simulink model "adaptive_mpc_simulink"  (R2019a)
settings: Solver=VariableStepAuto  StartTime=0.0  StopTime=10.0  RelTol=1e-3
libraries: mpclib x1
settings Model: Creator=alexh  LastModifiedBy=alexh

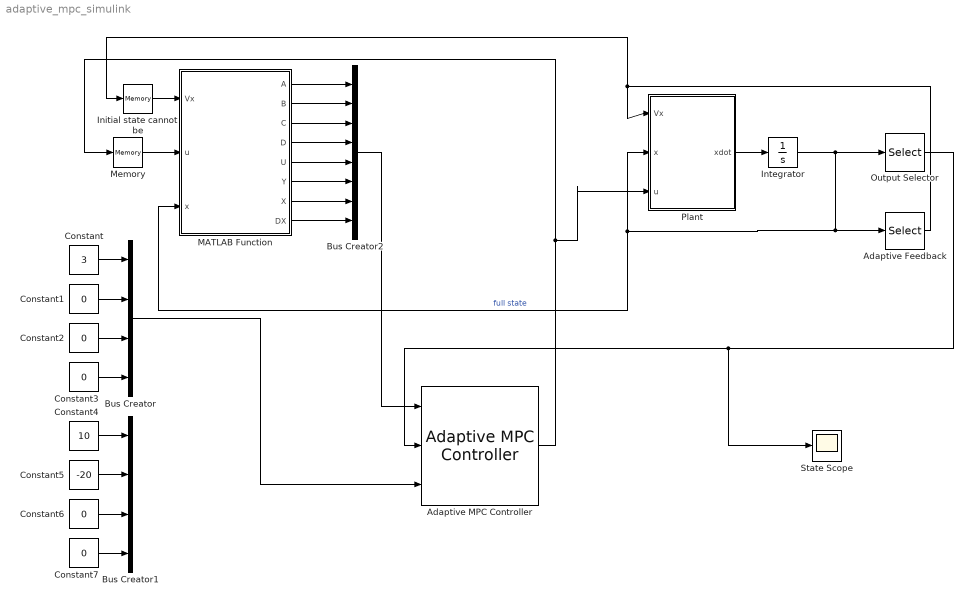
== system adaptive_mpc_simulink ==
  Adaptive Feedback : Selector  InputPortWidth=6  IndexOptions=Index vector (dialog)  Indices=[6]  OutputSizes=1
  Adaptive MPC Controller : mpclib/Adaptive MPC Controller  SCDEnableBlockLinearizationSpecification=on  mpcobj=mpc1_1_C  enable_value=0  updateMPCinCallerWorkspace=on  md_inport=off  mv_inport=off  uref_inport=off  return_cost=off  return_mvseq=off  return_qpstatus=off  return_xseq=off  return_state=off  return_ovseq=off  state_inport=off  isltv_plant=off  umin_inport=off  umax_inport=off  ymin_inport=off  ymax_inport=off  cc_inport=off  ywt_inport=off  uwt_inport=off  duwt_inport=off  rhoeps_inport=off  pm_inport=off  MaximumP=10  HorizonChoice=FixedHorizon  BlockDataType=double  SampleTimeInherited=off  switch_inport=off
      settings: SourceProductName=MATLAB Runtime - Model Predictive Control Toolbox Addin  SourceProductBaseCode=Missing
  Bus Creator : BusCreator  Inputs=4
  Bus Creator1 : BusCreator  Inputs=4
  Bus Creator2 : BusCreator  Inputs=8
  Constant : Constant  Value=3
  Constant{1..3,6..7} (5 alike) : Constant  Value=0
  Constant4 : Constant  Value=10
  Constant5 : Constant  Value=-20
  "Initial state cannot be " : Memory  InitialCondition=1
  Integrator : Integrator  ContinuousStateAttributes='vehicleState'
  MATLAB Function : MATLAB Function  TreatAsAtomicUnit=on
  Memory : Memory
  Output Selector : Selector  InputPortWidth=6  IndexOptions=Index vector (dialog)  Indices=[1 2 3 6]  OutputSizes=1
  Plant : MATLAB Function  TreatAsAtomicUnit=on
  State Scope : Scope
  wires:
  Adaptive MPC Controller/1 -> Memory/1, Plant/3(u)
  Plant/1(xdot) -> Integrator/1
  Integrator/1 -> Output Selector/1, Plant/2(x), MATLAB Function/3(x), Adaptive Feedback/1  "full state"
  Output Selector/1 -> State Scope/1, Adaptive MPC Controller/2
  Constant/1 -> Bus Creator/1
  Constant1/1 -> Bus Creator/2
  Constant2/1 -> Bus Creator/3
  Constant3/1 -> Bus Creator/4
  Constant7/1 -> Bus Creator1/4
  Constant6/1 -> Bus Creator1/3
  Constant5/1 -> Bus Creator1/2
  Constant4/1 -> Bus Creator1/1
  Bus Creator/1 -> Adaptive MPC Controller/3
  MATLAB Function/8(DX) -> Bus Creator2/8
  MATLAB Function/1(A) -> Bus Creator2/1
  MATLAB Function/2(B) -> Bus Creator2/2
  MATLAB Function/3(C) -> Bus Creator2/3
  MATLAB Function/4(D) -> Bus Creator2/4
  MATLAB Function/5(U) -> Bus Creator2/5
  MATLAB Function/6(Y) -> Bus Creator2/6
  MATLAB Function/7(X) -> Bus Creator2/7
  Bus Creator2/1 -> Adaptive MPC Controller/1
  Memory/1 -> MATLAB Function/2(u)
  Adaptive Feedback/1 -> "Initial state cannot be "/1, Plant/1(Vx)
  "Initial state cannot be "/1 -> MATLAB Function/1(Vx)

== matlab function adaptive_mpc_simulink/MATLAB Function ==
  data: Vx input; u input; A output; x input; B output; C output; D output; U output; Y output; X output; DX output
function [A,B,C,D,U,Y,X,DX] = fcn(Vx,u,x)
% Sample time
Ts = 0.1;

% Vehicule Parameter set up, all placeholders
m = 50;     % Mass
lf = 1;     % Distance mass center/front wheel
lr = 1;     % Distance mass center/rear wheel
Cf = 19000; % Cornering Stiffness front
Cr = 33000; % Cornering Stiffness rear
Iz = 2800;  % Yaw Moment of Innertia?

if( Vx < 0.1)
    Vx = 0.1;
end

% Continuous-time model
Ac = [0, 0, -Vx, 0, -1, 1;   %  Very crude spaceholder calc for x pos
    0, 0, Vx, 0, 1, 0;
    0, 0, 0, 1, 0, 0;
    0, 0, 0, -(2*Cf*lf^2+2*Cr*lr^2)/Iz/Vx, -(2*Cf*lf-2*Cr*lr)/Iz/Vx, 0;
    0, 0, 0, -Vx-(2*Cf*lf-2*Cr*lr)/m/Vx, -(2*Cf+2*Cr)/m/Vx, 0;
    0, 0, 0, 0, 0, 0.9        % Very crude definition of speed
    ];

Bc = [0, 0, 0, 2*Cf*lf/Iz, 2*Cf/m, 0;    % Steering angle
    0, 0, 0, 0, 0, 1]';                 % acceleration/break

Cc = [1, 0, 0, 0, 0, 0;
    0, 1, 0, 0, 0, 0;
    0, 0, 1, 0, 0, 0;
    0, 0, 0, 0, 0, 1];

Dc = zeros(4,2);

% Generate discrete-time model
nx = size(Ac,1);
nu = size(Bc,2);
M = expm([[Ac Bc]*Ts; zeros(nu,nx+nu)]);
A = M(1:nx,1:nx);
B = M(1:nx,nx+1:nx+nu);
C = Cc;
D = Dc;

% Nominal conditions for discrete-time plant
X = x';
U = u';
Y = (C*x + D*u)';
DX = (A*x+B*u-x)';
DX = [0, 0, 0, 0, 0, 0];

% Should be 6x1
% A 6x6 x=6x1
% B 6x2 u=2x1

== matlab function adaptive_mpc_simulink/Plant ==
  data: Vx input; x input; u input; xdot output
function xdot = fcn(Vx, x, u)

% Vehicule Parameter set up
m = 50;     % Mass
lf = 1;     % Distance mass center/front wheel
lr = 1;     % Distance mass center/rear wheel
Cf = 19000; % Cornering Stiffness front
Cr = 33000; % Cornering Stiffness rear
Iz = 2800;  % Yaw Moment of Innertia?

if (Vx < 0.01) 
    Vx = 0.01
end

% Continuous-time model
A = [0, 0, -Vx, 0, -1, 1;  
    %  Very crude spaceholder calc for x pos
    0, 0, Vx, 0, 1, 0;
    0, 0, 0, 1, 0, 0;
    0, 0, 0, -(2*Cf*lf^2+2*Cr*lr^2)/Iz/Vx, -(2*Cf*lf-2*Cr*lr)/Iz/Vx, 0;
    0, 0, 0, -Vx-(2*Cf*lf-2*Cr*lr)/m/Vx, -(2*Cf+2*Cr)/m/Vx, 0;
    0, 0, 0, 0, 0, -.1        % Very crude definition of speed
    ];

B = [0, 0, 0, 2*Cf*lf/Iz, 2*Cf/m, 0;    % Steering angle
    0, 0, 0, 0, 0, 1]';                 % acceleration/break

xdot = A*x + B*u;
